simulink model "Task1_simulink"  (R2026a)
settings: Solver=VariableStepAuto

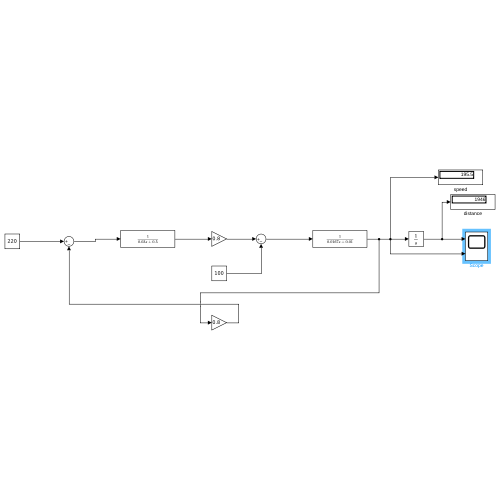
[thumbnail: Simulink's stored preview of the top-level diagram]
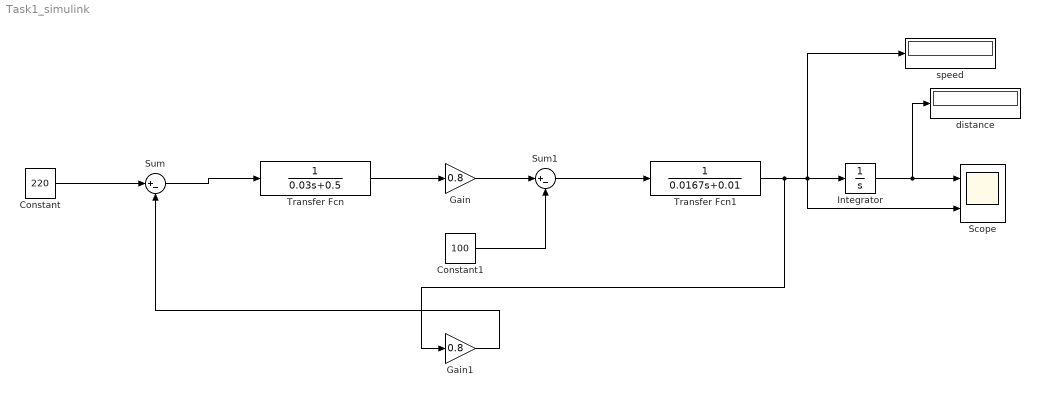
== system Task1_simulink ==
  Constant : Constant  Value=220
  Constant1 : Constant  Value=100
  Gain : Gain  Gain=0.8
  Gain1 : Gain  Gain=0.8
  Integrator : Integrator
  Scope : Scope  NumInputPorts=2
      settings: ActiveDisplayYMinimum=-294.06153860848713  ActiveDisplayYMaximum=2195.1303478773066
  Sum : Sum  Inputs=|+-
  Sum1 : Sum  Inputs=|+-
  Transfer Fcn : TransferFcn  Denominator=[0.03 0.5]
  Transfer Fcn1 : TransferFcn  Denominator=[0.0167 0.01]
  distance : Display
  speed : Display
  wires:
  Constant/1 -> Sum/1
  Sum/1 -> Transfer Fcn/1
  Transfer Fcn/1 -> Gain/1
  Gain/1 -> Sum1/1
  Constant1/1 -> Sum1/2
  Sum1/1 -> Transfer Fcn1/1
  Gain1/1 -> Sum/2
  Integrator/1 -> distance/1, Scope/1
  Transfer Fcn1/1 -> Scope/2, speed/1, Integrator/1, Gain1/1
